simulink model "zero_input_pole_placement"  (R2024a)
settings: Solver=VariableStepAuto  StartTime=0.0  StopTime=30  RelTol=1e-3
values from neighbouring files (symbols this model uses):
  A = [-1.7, -0.25, 0 ... (first row only)    [main.m]
  B = [7, 0 ... (first row only)    [main.m]
  K = real(R \ B' * P)    [LQR_own.m]    (also in decoupling.m = Bstar\C_star; main.m = real(inv(R)*B_bar'*P); pole_placement.m = Kbar*T)
  x0 = [1 100 200]'    [main.m]
settings Model: Creator=chint  LastModifiedBy=chint

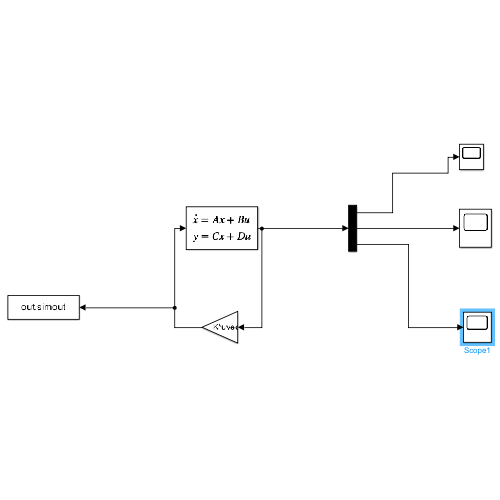
[thumbnail: Simulink's stored preview of the top-level diagram]
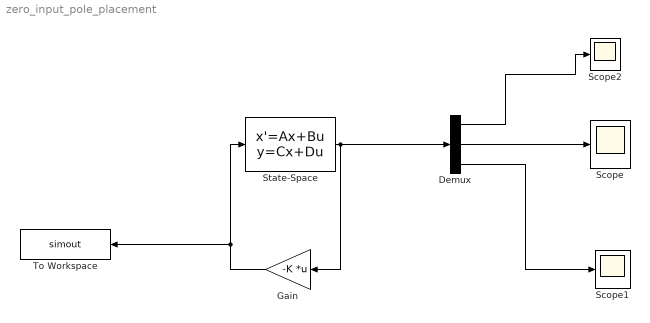
== system zero_input_pole_placement ==
  Demux : Demux  Outputs=3
  Gain : Gain  Gain=-K  Multiplication=Matrix(K*u) (u vector)
  Scope : Scope
  Scope1 : Scope
  Scope2 : Scope
  State-Space : StateSpace  A=A  B=B  C=eye(3)  D=[0 0; 0 0; 0 0]  InitialCondition=x0
  To Workspace : ToWorkspace  VariableName=simout  SaveFormat=Timeseries  SampleTime=-1
  wires:
  State-Space/1 -> Gain/1, Demux/1
  Gain/1 -> To Workspace/1, State-Space/1
  Demux/1 -> Scope2/1
  Demux/2 -> Scope/1
  Demux/3 -> Scope1/1
